simulink model "MTF"  (R2021a)
settings: Solver=VariableStepAuto  StartTime=0.0  StopTime=10.0  RelTol=1e-3
undefined symbols (not defined in the file or in its folder): B, C, D, E, Sh, Sv
settings Model: Creator=brianlesko  LastModifiedBy=brianlesko
settings DataIOCC: ReturnWorkspaceOutputs=off

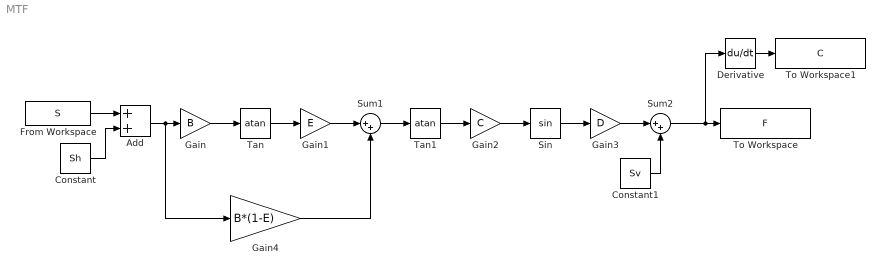
== system MTF ==
  Add : Sum
  Constant : Constant  Value=Sh
  Constant1 : Constant  Value=Sv
  Derivative : Derivative
  From Workspace : FromWorkspace  VariableName=S
  Gain : Gain  Gain=B
  Gain1 : Gain  Gain=E
  Gain2 : Gain  Gain=C
  Gain3 : Gain  Gain=D
  Gain4 : Gain  Gain=B*(1-E)
  Sin : Trigonometry
  Sum1 : Sum  Inputs=|++
  Sum2 : Sum  Inputs=|++
  Tan : Trigonometry  Operator=atan
  Tan1 : Trigonometry  Operator=atan
  To Workspace : ToWorkspace  VariableName=F  SampleTime=-1
      settings: MaxDataPoints=1
  To Workspace1 : ToWorkspace  VariableName=C  SaveFormat=Timeseries  SampleTime=-1
  wires:
  Constant/1 -> Add/2
  From Workspace/1 -> Add/1
  Add/1 -> Gain4/1, Gain/1
  Gain/1 -> Tan/1
  Tan/1 -> Gain1/1
  Gain1/1 -> Sum1/1
  Sum1/1 -> Tan1/1
  Tan1/1 -> Gain2/1
  Gain2/1 -> Sin/1
  Sin/1 -> Gain3/1
  Gain3/1 -> Sum2/1
  Sum2/1 -> Derivative/1, To Workspace/1
  Constant1/1 -> Sum2/2
  Gain4/1 -> Sum1/2
  Derivative/1 -> To Workspace1/1
